simulink model "tilt_telescopic_switch"  (R2020b)
settings: Solver=VariableStepAuto  StartTime=0.0  StopTime=inf  RelTol=1e-3
undefined symbols (not defined in the file): k_Switch_Debounce_Time, k_Switch_Release_Time, k_Switch_Stuck_Time, Tele_Input, Tilt_Input
libraries: simulink x4
settings Model: DataDictionary=tilt_telescopic_switch_DD.sldd  EnableAccessToBaseWorkspace=off  Creator=Jayesh Patil  LastModifiedBy=Jayesh Patil

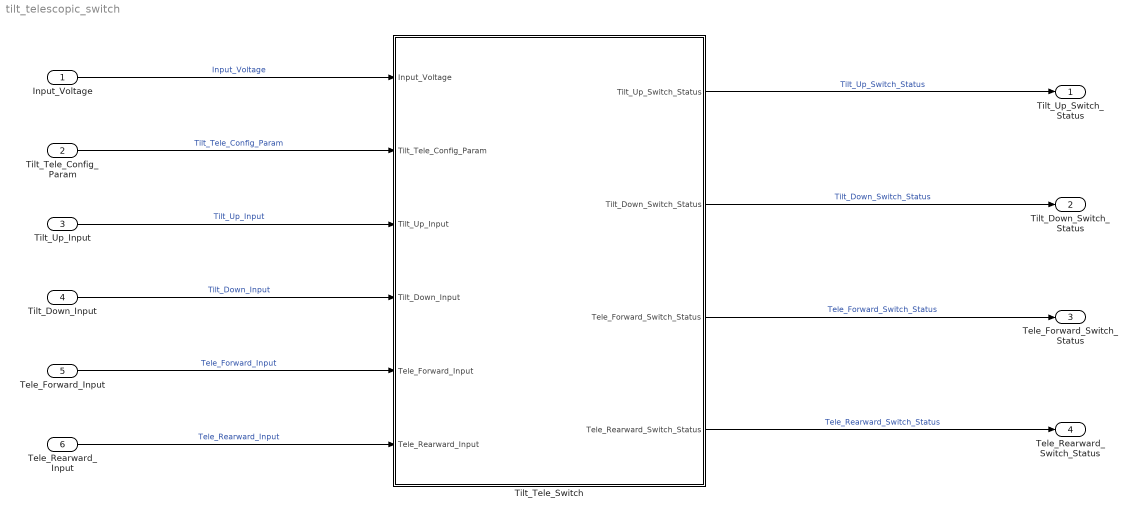
== system tilt_telescopic_switch ==
  Input_Voltage : Inport
  Tilt_Tele_Config_Param : Inport  Port=2
  Tilt_Up_Input : Inport  Port=3
  Tilt_Down_Input : Inport  Port=4
  Tele_Forward_Input : Inport  Port=5
  Tele_Rearward_Input : Inport  Port=6
  Tilt_Tele_Switch : Subsystem
  Tilt_Up_Switch_Status : Outport
  Tilt_Down_Switch_Status : Outport  Port=2
  Tele_Forward_Switch_Status : Outport  Port=3
  Tele_Rearward_Switch_Status : Outport  Port=4
  wires:
  Tele_Rearward_Input/1 -> Tilt_Tele_Switch/6(Tele_Rearward_Input)  "Tele_Rearward_Input"
  Tele_Forward_Input/1 -> Tilt_Tele_Switch/5(Tele_Forward_Input)  "Tele_Forward_Input"
  Tilt_Down_Input/1 -> Tilt_Tele_Switch/4(Tilt_Down_Input)  "Tilt_Down_Input"
  Tilt_Up_Input/1 -> Tilt_Tele_Switch/3(Tilt_Up_Input)  "Tilt_Up_Input"
  Tilt_Tele_Config_Param/1 -> Tilt_Tele_Switch/2(Tilt_Tele_Config_Param)  "Tilt_Tele_Config_Param"
  Input_Voltage/1 -> Tilt_Tele_Switch/1(Input_Voltage)  "Input_Voltage"
  Tilt_Tele_Switch/1(Tilt_Up_Switch_Status) -> Tilt_Up_Switch_Status/1  "Tilt_Up_Switch_Status"
  Tilt_Tele_Switch/2(Tilt_Down_Switch_Status) -> Tilt_Down_Switch_Status/1  "Tilt_Down_Switch_Status"
  Tilt_Tele_Switch/4(Tele_Rearward_Switch_Status) -> Tele_Rearward_Switch_Status/1  "Tele_Rearward_Switch_Status"
  Tilt_Tele_Switch/3(Tele_Forward_Switch_Status) -> Tele_Forward_Switch_Status/1  "Tele_Forward_Switch_Status"

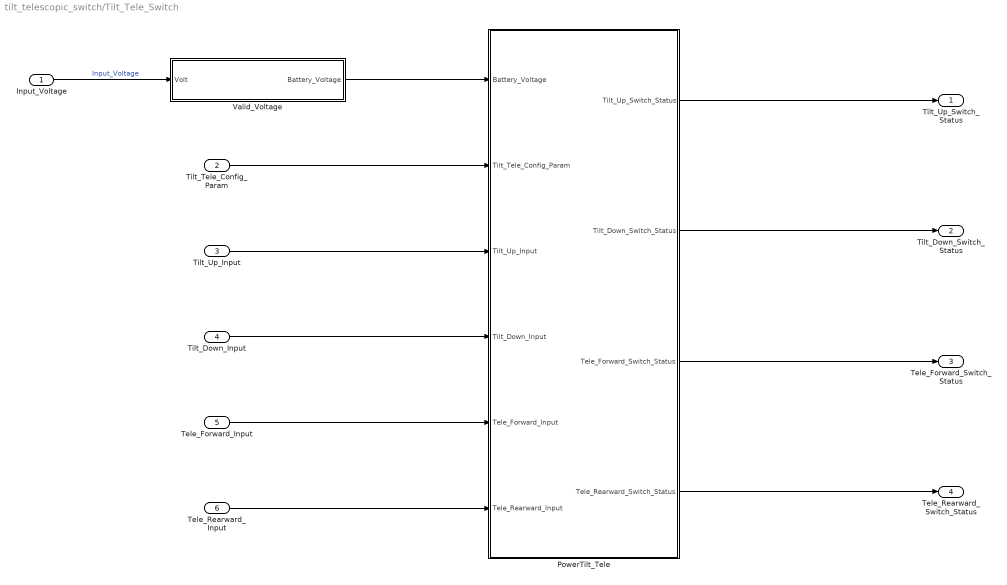
== system tilt_telescopic_switch/Tilt_Tele_Switch ==
  Input_Voltage : Inport
  Tilt_Tele_Config_Param : Inport  Port=2
  Tilt_Up_Input : Inport  Port=3
  Tilt_Down_Input : Inport  Port=4
  Tele_Forward_Input : Inport  Port=5
  Tele_Rearward_Input : Inport  Port=6
  PowerTilt_Tele : Subsystem
  Valid_Voltage : Subsystem
  Tilt_Up_Switch_Status : Outport
  Tilt_Down_Switch_Status : Outport  Port=2
  Tele_Forward_Switch_Status : Outport  Port=3
  Tele_Rearward_Switch_Status : Outport  Port=4
  wires:
  Input_Voltage/1 -> Valid_Voltage/1(Volt)  "Input_Voltage"
  Valid_Voltage/1(Battery_Voltage) -> PowerTilt_Tele/1(Battery_Voltage)
  Tilt_Tele_Config_Param/1 -> PowerTilt_Tele/2(Tilt_Tele_Config_Param)
  Tilt_Up_Input/1 -> PowerTilt_Tele/3(Tilt_Up_Input)
  Tilt_Down_Input/1 -> PowerTilt_Tele/4(Tilt_Down_Input)
  Tele_Forward_Input/1 -> PowerTilt_Tele/5(Tele_Forward_Input)
  Tele_Rearward_Input/1 -> PowerTilt_Tele/6(Tele_Rearward_Input)
  PowerTilt_Tele/1(Tilt_Up_Switch_Status) -> Tilt_Up_Switch_Status/1
  PowerTilt_Tele/3(Tele_Forward_Switch_Status) -> Tele_Forward_Switch_Status/1
  PowerTilt_Tele/4(Tele_Rearward_Switch_Status) -> Tele_Rearward_Switch_Status/1
  PowerTilt_Tele/2(Tilt_Down_Switch_Status) -> Tilt_Down_Switch_Status/1

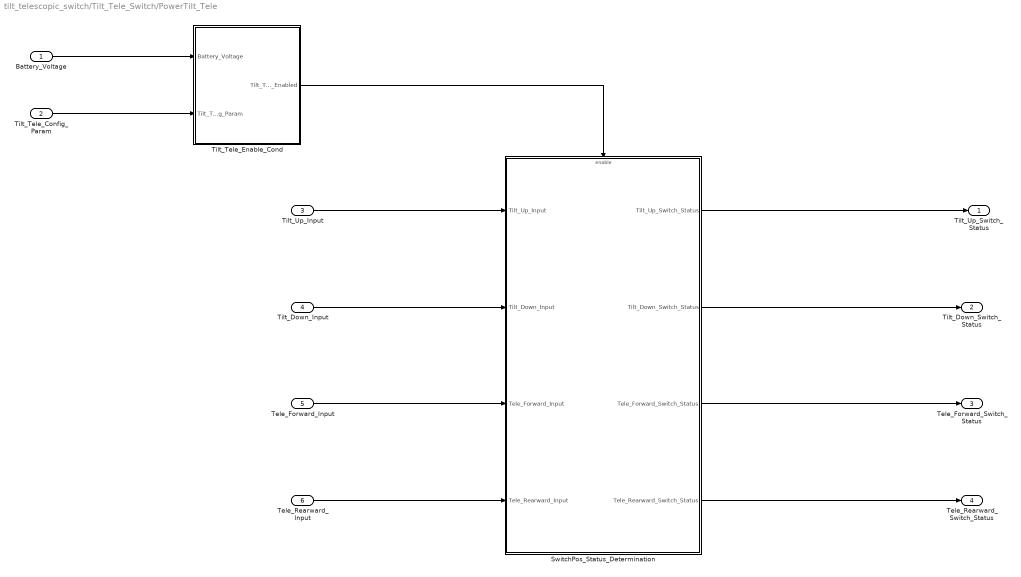
== system tilt_telescopic_switch/Tilt_Tele_Switch/PowerTilt_Tele ==
  Battery_Voltage : Inport
  Tilt_Tele_Config_Param : Inport  Port=2
  Tilt_Up_Input : Inport  Port=3
  Tilt_Down_Input : Inport  Port=4
  Tele_Forward_Input : Inport  Port=5
  Tele_Rearward_Input : Inport  Port=6
  SwitchPos_Status_Determination : Subsystem
  Tilt_Tele_Enable_Cond : Subsystem
  Tilt_Up_Switch_Status : Outport
  Tilt_Down_Switch_Status : Outport  Port=2
  Tele_Forward_Switch_Status : Outport  Port=3
  Tele_Rearward_Switch_Status : Outport  Port=4
  wires:
  Battery_Voltage/1 -> Tilt_Tele_Enable_Cond/1(Battery_Voltage)
  Tilt_Tele_Config_Param/1 -> Tilt_Tele_Enable_Cond/2(Tilt_Tele_Config_Param)
  Tilt_Up_Input/1 -> SwitchPos_Status_Determination/1(Tilt_Up_Input)
  Tilt_Down_Input/1 -> SwitchPos_Status_Determination/2(Tilt_Down_Input)
  Tele_Forward_Input/1 -> SwitchPos_Status_Determination/3(Tele_Forward_Input)
  Tele_Rearward_Input/1 -> SwitchPos_Status_Determination/4(Tele_Rearward_Input)
  SwitchPos_Status_Determination/1(Tilt_Up_Switch_Status) -> Tilt_Up_Switch_Status/1
  SwitchPos_Status_Determination/2(Tilt_Down_Switch_Status) -> Tilt_Down_Switch_Status/1
  SwitchPos_Status_Determination/3(Tele_Forward_Switch_Status) -> Tele_Forward_Switch_Status/1
  SwitchPos_Status_Determination/4(Tele_Rearward_Switch_Status) -> Tele_Rearward_Switch_Status/1
  Tilt_Tele_Enable_Cond/1(Tilt_Tele_Enabled) -> SwitchPos_Status_Determination/Enable

== system tilt_telescopic_switch/Tilt_Tele_Switch/Valid_Voltage ==
  Volt : Inport
  AND : Logic  AllPortsSameDT=off  OutDataTypeStr=boolean
  Relational Operator : RelationalOperator  OutDataTypeStr=boolean  RndMeth=Simplest
  Relational Operator1 : RelationalOperator  Operator=<=  OutDataTypeStr=boolean  RndMeth=Simplest
  VMax : Constant  Value=20  OutDataTypeStr=uint8
  VMin : Constant  Value=10  OutDataTypeStr=uint8
  Battery_Voltage : Outport
  wires:
  Volt/1 -> Relational Operator1/1, Relational Operator/1
  VMin/1 -> Relational Operator/2  "VMin"
  VMax/1 -> Relational Operator1/2  "VMax"
  AND/1 -> Battery_Voltage/1  "Battery_Voltage"
  Relational Operator/1 -> AND/1  "MinVolt"
  Relational Operator1/1 -> AND/2  "MaxVolt"

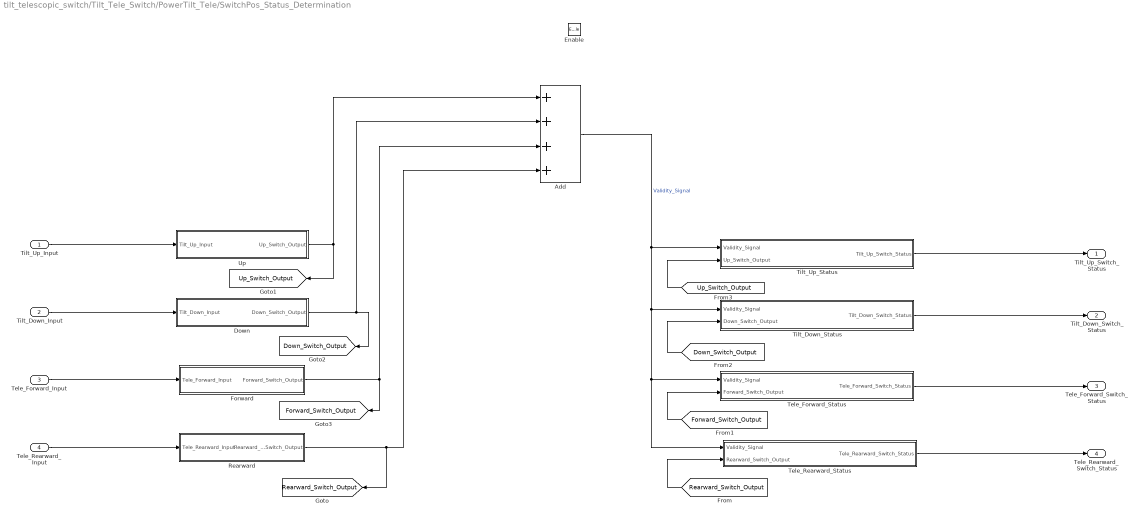
== system tilt_telescopic_switch/Tilt_Tele_Switch/PowerTilt_Tele/SwitchPos_Status_Determination ==
  Tilt_Up_Input : Inport
  Tilt_Down_Input : Inport  Port=2
  Tele_Forward_Input : Inport  Port=3
  Tele_Rearward_Input : Inport  Port=4
  Enable : EnablePort
  Add : Sum  Inputs=++++
  Down : Subsystem
  Forward : Subsystem
  Rearward : Subsystem
  Tele_Forward_Status : Subsystem
  Tele_Rearward_Status : Subsystem
  Tilt_Down_Status : Subsystem
  Tilt_Up_Status : Subsystem
  Up : Subsystem
  Tilt_Up_Switch_Status : Outport
  Tilt_Down_Switch_Status : Outport  Port=2
  Tele_Forward_Switch_Status : Outport  Port=3
  Tele_Rearward_Switch_Status : Outport  Port=4
  tag scope: Down_Switch_Output=global, Forward_Switch_Output=global, Rearward_Switch_Output=global, Up_Switch_Output=global
  wires:
  Up/1(Up_Switch_Output) -> [Up_Switch_Output], Add/1
  Down/1(Down_Switch_Output) -> [Down_Switch_Output], Add/2
  Forward/1(Forward_Switch_Output) -> [Forward_Switch_Output], Add/3
  Rearward/1(Rearward_Switch_Output) -> [Rearward_Switch_Output], Add/4
  Tilt_Up_Input/1 -> Up/1(Tilt_Up_Input)
  Tilt_Down_Input/1 -> Down/1(Tilt_Down_Input)
  Tele_Forward_Input/1 -> Forward/1(Tele_Forward_Input)
  Tele_Rearward_Input/1 -> Rearward/1(Tele_Rearward_Input)
  Tilt_Up_Status/1(Tilt_Up_Switch_Status) -> Tilt_Up_Switch_Status/1
  Tilt_Down_Status/1(Tilt_Down_Switch_Status) -> Tilt_Down_Switch_Status/1
  Tele_Forward_Status/1(Tele_Forward_Switch_Status) -> Tele_Forward_Switch_Status/1
  Tele_Rearward_Status/1(Tele_Rearward_Switch_Status) -> Tele_Rearward_Switch_Status/1
  Add/1 -> Tilt_Up_Status/1(Validity_Signal), Tele_Rearward_Status/1(Validity_Signal), Tele_Forward_Status/1(Validity_Signal), Tilt_Down_Status/1(Validity_Signal)  "Validity_Signal"
  [Rearward_Switch_Output] -> Tele_Rearward_Status/2(Rearward_Switch_Output)
  [Forward_Switch_Output] -> Tele_Forward_Status/2(Forward_Switch_Output)
  [Down_Switch_Output] -> Tilt_Down_Status/2(Down_Switch_Output)
  [Up_Switch_Output] -> Tilt_Up_Status/2(Up_Switch_Output)

== system tilt_telescopic_switch/Tilt_Tele_Switch/PowerTilt_Tele/Tilt_Tele_Enable_Cond ==
  Battery_Voltage : Inport
  Tilt_Tele_Config_Param : Inport  Port=2
  AND : Logic  AllPortsSameDT=off  OutDataTypeStr=boolean
  Tilt_Tele_Enabled : Outport
  wires:
  Tilt_Tele_Config_Param/1 -> AND/2
  Battery_Voltage/1 -> AND/1
  AND/1 -> Tilt_Tele_Enabled/1  "Tilt_Tele_Enabled"

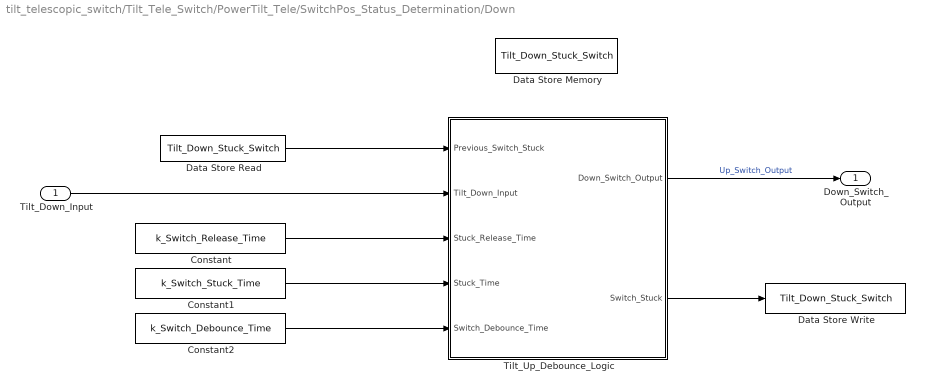
== system tilt_telescopic_switch/Tilt_Tele_Switch/PowerTilt_Tele/SwitchPos_Status_Determination/Down ==
  Tilt_Down_Input : Inport
  Constant : Constant  Value=k_Switch_Release_Time
  Constant1 : Constant  Value=k_Switch_Stuck_Time
  Constant2 : Constant  Value=k_Switch_Debounce_Time
  Data Store Memory : DataStoreMemory  DataStoreName=Tilt_Down_Stuck_Switch  ReadBeforeWriteMsg=warning  WriteAfterWriteMsg=warning  WriteAfterReadMsg=warning  ShowAdditionalParam=off  StateMustResolveToSignalObject=on
  Data Store Read : DataStoreRead  DataStoreName=Tilt_Down_Stuck_Switch
  Data Store Write : DataStoreWrite  DataStoreName=Tilt_Down_Stuck_Switch
  Tilt_Up_Debounce_Logic : Stateflow chart  TreatAsAtomicUnit=on
  Down_Switch_Output : Outport
  wires:
  Constant2/1 -> Tilt_Up_Debounce_Logic/5(Switch_Debounce_Time)
  Constant1/1 -> Tilt_Up_Debounce_Logic/4(Stuck_Time)
  Constant/1 -> Tilt_Up_Debounce_Logic/3(Stuck_Release_Time)
  Tilt_Down_Input/1 -> Tilt_Up_Debounce_Logic/2(Tilt_Down_Input)
  Tilt_Up_Debounce_Logic/1(Down_Switch_Output) -> Down_Switch_Output/1  "Up_Switch_Output"
  Tilt_Up_Debounce_Logic/2(Switch_Stuck) -> Data Store Write/1
  Data Store Read/1 -> Tilt_Up_Debounce_Logic/1(Previous_Switch_Stuck)

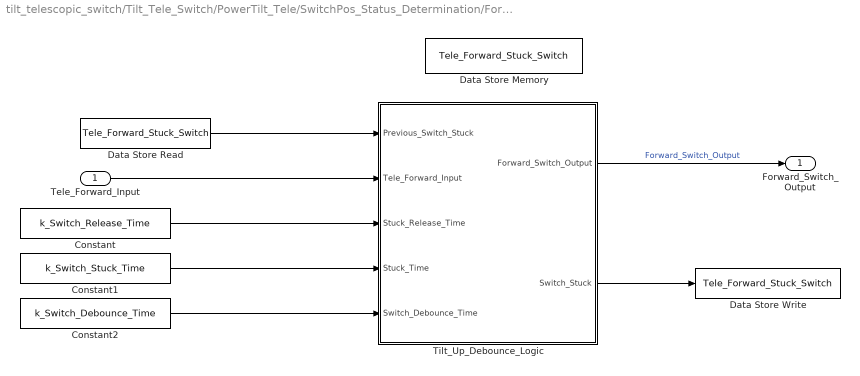
== system tilt_telescopic_switch/Tilt_Tele_Switch/PowerTilt_Tele/SwitchPos_Status_Determination/Forward ==
  Tele_Forward_Input : Inport
  Constant : Constant  Value=k_Switch_Release_Time
  Constant1 : Constant  Value=k_Switch_Stuck_Time
  Constant2 : Constant  Value=k_Switch_Debounce_Time
  Data Store Memory : DataStoreMemory  DataStoreName=Tele_Forward_Stuck_Switch  ReadBeforeWriteMsg=warning  WriteAfterWriteMsg=warning  WriteAfterReadMsg=warning  ShowAdditionalParam=off  StateMustResolveToSignalObject=on
  Data Store Read : DataStoreRead  DataStoreName=Tele_Forward_Stuck_Switch
  Data Store Write : DataStoreWrite  DataStoreName=Tele_Forward_Stuck_Switch
  Tilt_Up_Debounce_Logic : Stateflow chart  TreatAsAtomicUnit=on
  Forward_Switch_Output : Outport
  wires:
  Constant2/1 -> Tilt_Up_Debounce_Logic/5(Switch_Debounce_Time)
  Constant1/1 -> Tilt_Up_Debounce_Logic/4(Stuck_Time)
  Constant/1 -> Tilt_Up_Debounce_Logic/3(Stuck_Release_Time)
  Tele_Forward_Input/1 -> Tilt_Up_Debounce_Logic/2(Tele_Forward_Input)
  Tilt_Up_Debounce_Logic/1(Forward_Switch_Output) -> Forward_Switch_Output/1  "Forward_Switch_Output"
  Data Store Read/1 -> Tilt_Up_Debounce_Logic/1(Previous_Switch_Stuck)
  Tilt_Up_Debounce_Logic/2(Switch_Stuck) -> Data Store Write/1

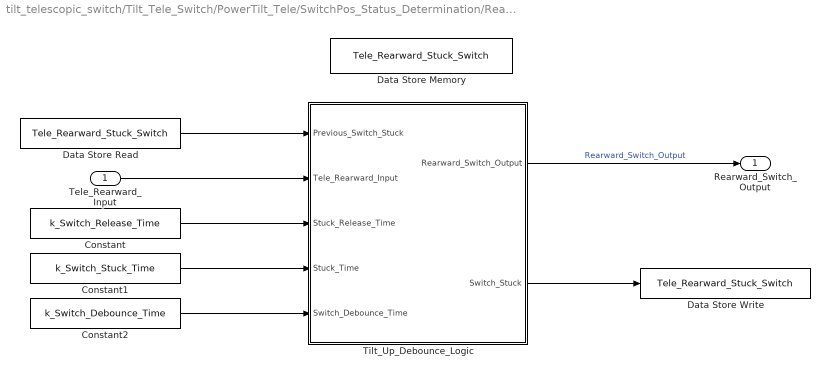
== system tilt_telescopic_switch/Tilt_Tele_Switch/PowerTilt_Tele/SwitchPos_Status_Determination/Rearward ==
  Tele_Rearward_Input : Inport
  Constant : Constant  Value=k_Switch_Release_Time
  Constant1 : Constant  Value=k_Switch_Stuck_Time
  Constant2 : Constant  Value=k_Switch_Debounce_Time
  Data Store Memory : DataStoreMemory  DataStoreName=Tele_Rearward_Stuck_Switch  ReadBeforeWriteMsg=warning  WriteAfterWriteMsg=warning  WriteAfterReadMsg=warning  ShowAdditionalParam=off  StateMustResolveToSignalObject=on
  Data Store Read : DataStoreRead  DataStoreName=Tele_Rearward_Stuck_Switch
  Data Store Write : DataStoreWrite  DataStoreName=Tele_Rearward_Stuck_Switch
  Tilt_Up_Debounce_Logic : Stateflow chart  TreatAsAtomicUnit=on
  Rearward_Switch_Output : Outport
  wires:
  Tilt_Up_Debounce_Logic/2(Switch_Stuck) -> Data Store Write/1
  Data Store Read/1 -> Tilt_Up_Debounce_Logic/1(Previous_Switch_Stuck)
  Constant2/1 -> Tilt_Up_Debounce_Logic/5(Switch_Debounce_Time)
  Constant1/1 -> Tilt_Up_Debounce_Logic/4(Stuck_Time)
  Constant/1 -> Tilt_Up_Debounce_Logic/3(Stuck_Release_Time)
  Tele_Rearward_Input/1 -> Tilt_Up_Debounce_Logic/2(Tele_Rearward_Input)
  Tilt_Up_Debounce_Logic/1(Rearward_Switch_Output) -> Rearward_Switch_Output/1  "Rearward_Switch_Output"

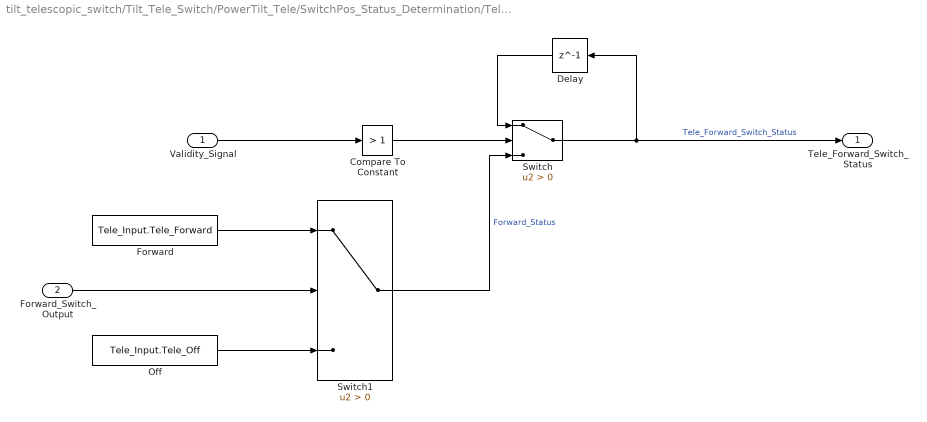
== system tilt_telescopic_switch/Tilt_Tele_Switch/PowerTilt_Tele/SwitchPos_Status_Determination/Tele_Forward_Status ==
  Validity_Signal : Inport
  Forward_Switch_Output : Inport  Port=2
  Compare To Constant : simulink/Logic and Bit Operations/Compare To Constant  relop=>  const=1  OutDataTypeStr=boolean
  Delay : Delay  DelayLength=1  InitialCondition=Tele_Input.Tele_Off  StateName=Tele_Forward_Switch_Status_Delay  StateMustResolveToSignalObject=on
  Forward : Constant  Value=Tele_Input.Tele_Forward
  Off : Constant  Value=Tele_Input.Tele_Off
  Switch : Switch  Criteria=u2 > Threshold
  Switch1 : Switch  Criteria=u2 > Threshold
  Tele_Forward_Switch_Status : Outport
  wires:
  Switch1/1 -> Switch/3  "Forward_Status"
  Compare To Constant/1 -> Switch/2
  Delay/1 -> Switch/1
  Switch/1 -> Tele_Forward_Switch_Status/1, Delay/1  "Tele_Forward_Switch_Status"
  Forward_Switch_Output/1 -> Switch1/2
  Off/1 -> Switch1/3
  Validity_Signal/1 -> Compare To Constant/1
  Forward/1 -> Switch1/1

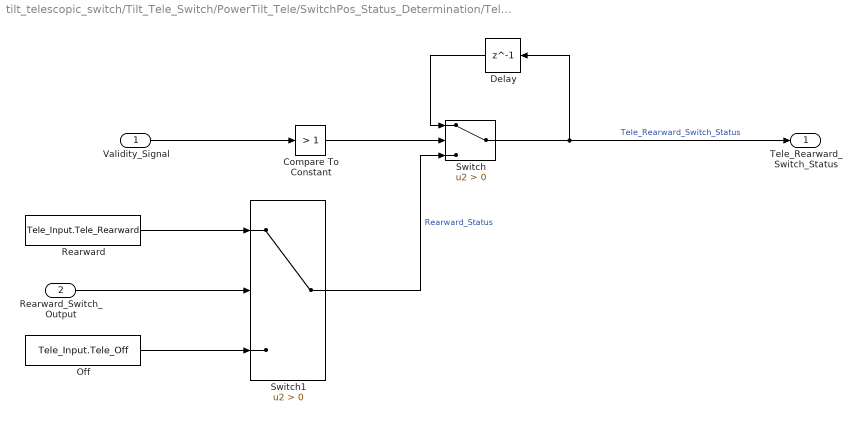
== system tilt_telescopic_switch/Tilt_Tele_Switch/PowerTilt_Tele/SwitchPos_Status_Determination/Tele_Rearward_Status ==
  Validity_Signal : Inport
  Rearward_Switch_Output : Inport  Port=2
  Compare To Constant : simulink/Logic and Bit Operations/Compare To Constant  relop=>  const=1  OutDataTypeStr=boolean
  Delay : Delay  DelayLength=1  InitialCondition=Tele_Input.Tele_Off  StateName=Tele_Rearward_Switch_Status_Delay  StateMustResolveToSignalObject=on
  Off : Constant  Value=Tele_Input.Tele_Off
  Rearward : Constant  Value=Tele_Input.Tele_Rearward
  Switch : Switch  Criteria=u2 > Threshold
  Switch1 : Switch  Criteria=u2 > Threshold
  Tele_Rearward_Switch_Status : Outport
  wires:
  Switch1/1 -> Switch/3  "Rearward_Status"
  Compare To Constant/1 -> Switch/2
  Delay/1 -> Switch/1
  Switch/1 -> Tele_Rearward_Switch_Status/1, Delay/1  "Tele_Rearward_Switch_Status"
  Rearward_Switch_Output/1 -> Switch1/2
  Off/1 -> Switch1/3
  Validity_Signal/1 -> Compare To Constant/1
  Rearward/1 -> Switch1/1

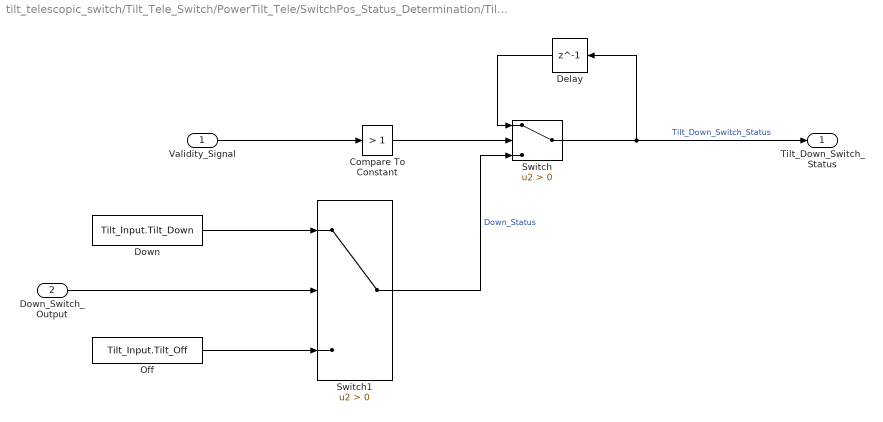
== system tilt_telescopic_switch/Tilt_Tele_Switch/PowerTilt_Tele/SwitchPos_Status_Determination/Tilt_Down_Status ==
  Validity_Signal : Inport
  Down_Switch_Output : Inport  Port=2
  Compare To Constant : simulink/Logic and Bit Operations/Compare To Constant  relop=>  const=1  OutDataTypeStr=boolean
  Delay : Delay  DelayLength=1  InitialCondition=Tilt_Input.Tilt_Off  StateName=Tilt_Down_Switch_Status_Delay  StateMustResolveToSignalObject=on
  Down : Constant  Value=Tilt_Input.Tilt_Down
  Off : Constant  Value=Tilt_Input.Tilt_Off
  Switch : Switch  Criteria=u2 > Threshold
  Switch1 : Switch  Criteria=u2 > Threshold
  Tilt_Down_Switch_Status : Outport
  wires:
  Switch1/1 -> Switch/3  "Down_Status"
  Compare To Constant/1 -> Switch/2
  Delay/1 -> Switch/1
  Switch/1 -> Tilt_Down_Switch_Status/1, Delay/1  "Tilt_Down_Switch_Status"
  Down_Switch_Output/1 -> Switch1/2
  Off/1 -> Switch1/3
  Validity_Signal/1 -> Compare To Constant/1
  Down/1 -> Switch1/1

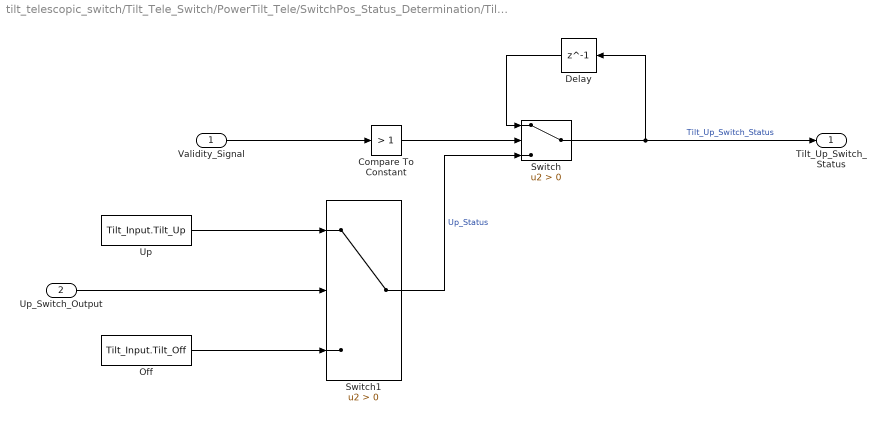
== system tilt_telescopic_switch/Tilt_Tele_Switch/PowerTilt_Tele/SwitchPos_Status_Determination/Tilt_Up_Status ==
  Validity_Signal : Inport
  Up_Switch_Output : Inport  Port=2
  Compare To Constant : simulink/Logic and Bit Operations/Compare To Constant  relop=>  const=1  OutDataTypeStr=boolean
  Delay : Delay  DelayLength=1  InitialCondition=Tilt_Input.Tilt_Off  StateName=Tilt_Up_Switch_Status_Delay  StateMustResolveToSignalObject=on
  Off : Constant  Value=Tilt_Input.Tilt_Off
  Switch : Switch  Criteria=u2 > Threshold
  Switch1 : Switch  Criteria=u2 > Threshold
  Up : Constant  Value=Tilt_Input.Tilt_Up
  Tilt_Up_Switch_Status : Outport
  wires:
  Compare To Constant/1 -> Switch/2
  Validity_Signal/1 -> Compare To Constant/1
  Switch/1 -> Delay/1, Tilt_Up_Switch_Status/1  "Tilt_Up_Switch_Status"
  Delay/1 -> Switch/1
  Up_Switch_Output/1 -> Switch1/2
  Up/1 -> Switch1/1
  Off/1 -> Switch1/3
  Switch1/1 -> Switch/3  "Up_Status"

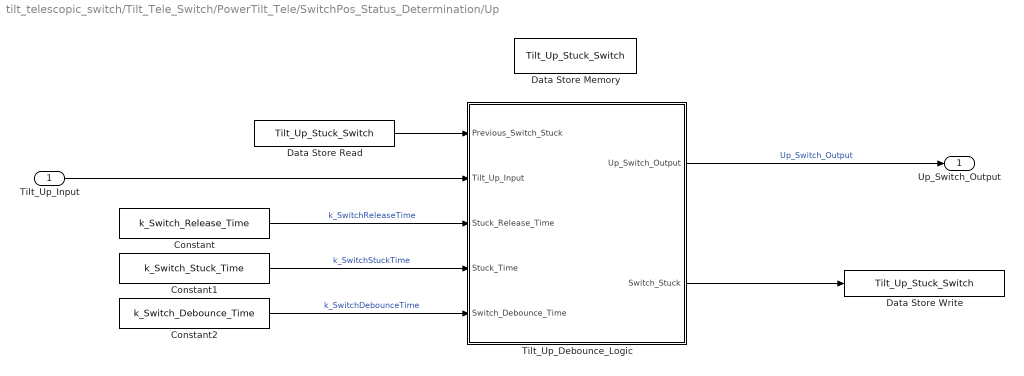
== system tilt_telescopic_switch/Tilt_Tele_Switch/PowerTilt_Tele/SwitchPos_Status_Determination/Up ==
  Tilt_Up_Input : Inport
  Constant : Constant  Value=k_Switch_Release_Time
  Constant1 : Constant  Value=k_Switch_Stuck_Time
  Constant2 : Constant  Value=k_Switch_Debounce_Time
  Data Store Memory : DataStoreMemory  DataStoreName=Tilt_Up_Stuck_Switch  ReadBeforeWriteMsg=warning  WriteAfterWriteMsg=warning  WriteAfterReadMsg=warning  ShowAdditionalParam=off  StateMustResolveToSignalObject=on
  Data Store Read : DataStoreRead  DataStoreName=Tilt_Up_Stuck_Switch
  Data Store Write : DataStoreWrite  DataStoreName=Tilt_Up_Stuck_Switch
  Tilt_Up_Debounce_Logic : Stateflow chart  TreatAsAtomicUnit=on
  Up_Switch_Output : Outport
  wires:
  Constant/1 -> Tilt_Up_Debounce_Logic/3(Stuck_Release_Time)  "k_SwitchReleaseTime"
  Constant1/1 -> Tilt_Up_Debounce_Logic/4(Stuck_Time)  "k_SwitchStuckTime"
  Constant2/1 -> Tilt_Up_Debounce_Logic/5(Switch_Debounce_Time)  "k_SwitchDebounceTime"
  Tilt_Up_Input/1 -> Tilt_Up_Debounce_Logic/2(Tilt_Up_Input)
  Tilt_Up_Debounce_Logic/1(Up_Switch_Output) -> Up_Switch_Output/1  "Up_Switch_Output"
  Data Store Read/1 -> Tilt_Up_Debounce_Logic/1(Previous_Switch_Stuck)
  Tilt_Up_Debounce_Logic/2(Switch_Stuck) -> Data Store Write/1

== stateflow chart tilt_telescopic_switch/Tilt_Tele_Switch/PowerTilt_Tele/SwitchPos_Status_Determination/Rearward/Tilt_Up_Debounce_Logic ==
  state Not_Pressed
    en:
    Rearward_Switch_Output = false;
  state Debounce
    state Off_Debounce
    state On_Debounce
  state Pressed
    en:
    Rearward_Switch_Output = true;
  state Off
  state Stuck_Wait
  state Stuck
    en:
    Rearward_Switch_Output = false;
    Switch_Stuck = true;
  (default) -> Not_Pressed
  Off -> Not_Pressed : [after(Stuck_Release_Time,sec)]
  Not_Pressed -> On_Debounce : [(Previous_Switch_Stuck==false)&&(Tele_Rearward_Input==true)]
  Pressed -> Off_Debounce [order 2]
  On_Debounce -> Pressed : [after(Switch_Debounce_Time,sec)]
  Stuck -> Off : [Tele_Rearward_Input==true]
  Pressed -> Stuck_Wait [order 1] : [after(Stuck_Time-Switch_Debounce_Time,sec)]
  Stuck_Wait -> Stuck : [Tele_Rearward_Input==true]
  data: Previous_Switch_Stuck input boolean; Tele_Rearward_Input input boolean; Stuck_Release_Time input uint8; Stuck_Time input uint8; Switch_Debounce_Time input uint8; Rearward_Switch_Output output boolean; Switch_Stuck output boolean

== stateflow chart tilt_telescopic_switch/Tilt_Tele_Switch/PowerTilt_Tele/SwitchPos_Status_Determination/Down/Tilt_Up_Debounce_Logic ==
  state Not_Pressed
    en:
    Down_Switch_Output = false;
  state Debounce
    state Off_Debounce
    state On_Debounce
  state Pressed
    en:
    Down_Switch_Output = true;
  state Off
  state Stuck_Wait
  state Stuck
    en:
    Down_Switch_Output = false;
    Switch_Stuck = true;
  (default) -> Not_Pressed
  Off -> Not_Pressed : [after(Stuck_Release_Time,sec)]
  Not_Pressed -> On_Debounce : [(Previous_Switch_Stuck==false)&&(Tilt_Down_Input==true)]
  Pressed -> Off_Debounce [order 2]
  On_Debounce -> Pressed : [after(Switch_Debounce_Time,sec)]
  Stuck -> Off : [Tilt_Down_Input==true]
  Pressed -> Stuck_Wait [order 1] : [after(Stuck_Time-Switch_Debounce_Time,sec)]
  Stuck_Wait -> Stuck : [Tilt_Down_Input==true]
  data: Previous_Switch_Stuck input boolean; Tilt_Down_Input input boolean; Stuck_Release_Time input uint8; Stuck_Time input uint8; Switch_Debounce_Time input uint8; Down_Switch_Output output boolean; Switch_Stuck output boolean

== stateflow chart tilt_telescopic_switch/Tilt_Tele_Switch/PowerTilt_Tele/SwitchPos_Status_Determination/Forward/Tilt_Up_Debounce_Logic ==
  state Not_Pressed
    en:
    Forward_Switch_Output = false;
  state Debounce
    state Off_Debounce
    state On_Debounce
  state Pressed
    en:
    Forward_Switch_Output = true;
  state Off
  state Stuck_Wait
  state Stuck
    en:
    Forward_Switch_Output = false;
    Switch_Stuck = true;
  (default) -> Not_Pressed
  Off -> Not_Pressed : [after(Stuck_Release_Time,sec)]
  Not_Pressed -> On_Debounce : [(Previous_Switch_Stuck==false)&&(Tele_Forward_Input==true)]
  Pressed -> Off_Debounce [order 2]
  On_Debounce -> Pressed : [after(Switch_Debounce_Time,sec)]
  Stuck -> Off : [Tele_Forward_Input==true]
  Pressed -> Stuck_Wait [order 1] : [after(Stuck_Time-Switch_Debounce_Time,sec)]
  Stuck_Wait -> Stuck : [Tele_Forward_Input==true]
  data: Previous_Switch_Stuck input boolean; Tele_Forward_Input input boolean; Stuck_Release_Time input uint8; Stuck_Time input uint8; Switch_Debounce_Time input uint8; Forward_Switch_Output output boolean; Switch_Stuck output boolean

== stateflow chart tilt_telescopic_switch/Tilt_Tele_Switch/PowerTilt_Tele/SwitchPos_Status_Determination/Up/Tilt_Up_Debounce_Logic ==
  state Not_Pressed
    en:
    Up_Switch_Output = false;
  state Debounce
    state Off_Debounce
    state On_Debounce
  state Pressed
    en:
    Up_Switch_Output = true;
  state Off
  state Stuck_Wait
  state Stuck
    en:
    Up_Switch_Output = false;
    Switch_Stuck = true;
  (default) -> Not_Pressed
  Off -> Not_Pressed : [after(Stuck_Release_Time,sec)]
  Not_Pressed -> On_Debounce : [(Previous_Switch_Stuck==false)&&(Tilt_Up_Input==true)]
  Pressed -> Off_Debounce [order 2]
  On_Debounce -> Pressed : [after(Switch_Debounce_Time,sec)]
  Stuck -> Off : [Tilt_Up_Input==true]
  Pressed -> Stuck_Wait [order 1] : [after(Stuck_Time-Switch_Debounce_Time,sec)]
  Stuck_Wait -> Stuck : [Tilt_Up_Input==true]
  data: Previous_Switch_Stuck input boolean; Tilt_Up_Input input boolean; Stuck_Release_Time input uint8; Stuck_Time input uint8; Switch_Debounce_Time input uint8; Up_Switch_Output output boolean; Switch_Stuck output boolean
